simulink model "Motor_1"  (Simulink 7.1)
settings: Solver=ode45  StartTime=0.0  StopTime=1  MaxStep=0.01  RelTol=1e-3
undefined symbols (not defined in the file): Ispez, J, L, R
settings Model: Creator=dep19025415  LastModifiedBy=dep19025415

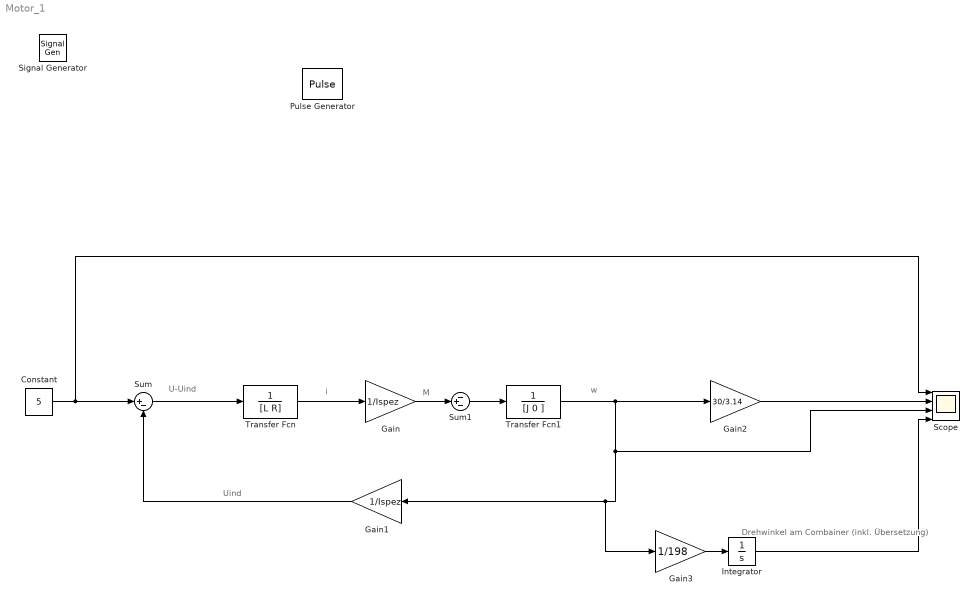
== system Motor_1 ==
  note: Uind
  note: U-Uind
  note: i
  note: M
  note: w
  note: Drehwinkel am Combainer
      |  (inkl. Übersetzung)
  Constant : Constant  Value=5  OutDataType=sfix(16)  OutScaling=2^0
  Gain : Gain  Gain=1/Ispez  ParameterDataType=sfix(16)  ParameterScaling=2^0  OutDataType=sfix(16)  OutScaling=2^0
  Gain1 : Gain  Orientation=left  Gain=1/Ispez  ParameterDataType=sfix(16)  ParameterScaling=2^0  OutDataType=sfix(16)  OutScaling=2^0
  Gain2 : Gain  Gain=30/3.14  ParameterDataType=sfix(16)  ParameterScaling=2^0  OutDataType=sfix(16)  OutScaling=2^0
  Gain3 : Gain  Gain=1/198  ParameterDataType=sfix(16)  ParameterScaling=2^0  OutDataType=sfix(16)  OutScaling=2^0
  Integrator : Integrator
  Pulse Generator : DiscretePulseGenerator  PulseType=Time based  Amplitude=8  Period=1  PulseWidth=2  SampleTime=0.1  VectorParams1D=off
  Scope : Scope  NumInputPorts=4
      settings: YMin=-10~0~-5~-5  YMax=10~5000~5~5
  Signal Generator : SignalGenerator
  Sum : Sum  Inputs=|+-  OutDataType=sfix(16)  OutScaling=2^0
  Sum1 : Sum  Inputs=-+-  OutDataType=sfix(16)  OutScaling=2^0
  Transfer Fcn : TransferFcn  Denominator=[L R]
  Transfer Fcn1 : TransferFcn  Denominator=[J 0 ]
  wires:
  Transfer Fcn/1 -> Gain/1
  Transfer Fcn1/1 -> Scope/3, Gain1/1, Gain3/1, Gain2/1
  Sum/1 -> Transfer Fcn/1
  Gain1/1 -> Sum/2
  Gain2/1 -> Scope/2
  Gain/1 -> Sum1/2
  Sum1/1 -> Transfer Fcn1/1
  Integrator/1 -> Scope/4
  Gain3/1 -> Integrator/1
  Constant/1 -> Sum/1, Scope/1
